simulink library "PES_CZ_FAW"  (Simulink 7.5)
settings: Solver=FixedStepDiscrete  StartTime=0.0  StopTime=10.0  FixedStep=0.01  MaxStep=0.01  RelTol=1e-3
undefined symbols (not defined in the file or in its folder): DiscIntNeverNeededParam, p_DRC_LoPsFilActPwr_s, p_DRC_LoPsFilPwrTi_s, p_DRC_LPFiltIC2_Tau_s, p_DRC_LPFiltIC2_Ts_s, p_DRC_LPFiltIC_Tau_s, p_DRC_LPFiltIC_Ts_s, Slope1, Slope2
libraries: BaseOperationLib_Browser x128, simulink x1
(part 2 of 2)

== system PES_CZ_FAW/Filters/LPFiltICEnRst/UD_EnResetIC ==
  u : Inport
  E : Inport  Port=2
  R : Inport  Port=3
  IC : Inport  Port=4
  Enable : BaseOperationLib_Browser/Signal Routing Changed/Switch  Criteria=u2 ~= 0  Threshold=0  OutMin=[]  OutMax=[]  OutDataType=fixdt(1,16,0)  OutScaling=[]  OutDataTypeStr=Inherit: Inherit via back propagation
  FixPt Data Type Duplicate1 : DataTypeDuplicate  NumInputPorts=4
  UD_Rst_IC : Subsystem
  y : Outport
  wires:
  UD_Rst_IC/1(y) -> y/1, Enable/3, FixPt Data Type Duplicate1/1
  R/1 -> UD_Rst_IC/2(R)
  Enable/1 -> UD_Rst_IC/1(u), FixPt Data Type Duplicate1/3
  u/1 -> Enable/1, FixPt Data Type Duplicate1/4
  IC/1 -> UD_Rst_IC/3(IC), FixPt Data Type Duplicate1/2
  E/1 -> Enable/2

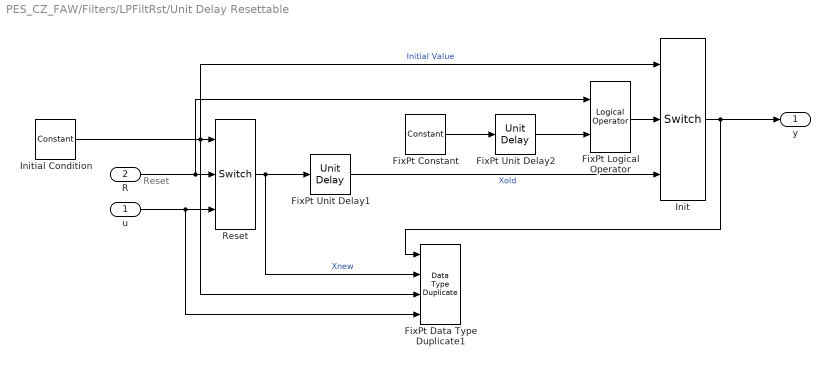
== system PES_CZ_FAW/Filters/LPFiltRst/Unit Delay Resettable ==
  note: Reset
  u : Inport
  R : Inport  Port=2
  FixPt Constant : BaseOperationLib_Browser/Sources&Sinks/Constant  Value=0  OutMin=[]  OutMax=[]  OutDataTypeMode=Specify via dialog  OutDataType=fixdt(0,8,0)  ConRadixGroup=Best Precision: Vector-wise  OutScaling=[]  OutDataTypeStr=fixdt(0,8,0)
  FixPt Data Type Duplicate1 : DataTypeDuplicate  NumInputPorts=4
  FixPt Logical Operator : BaseOperationLib_Browser/Logic Operations Changed/Logical Operator  Operator=OR  Inputs=2  AllPortsSameDT=off  OutDataTypeMode=Specify via dialog  LogicDataType=fixdt(0, 8)  OutDataTypeStr=fixdt(0, 8)
  FixPt Unit Delay1 : BaseOperationLib_Browser/Discrete Unchanged /Unit Delay  X0=0  SampleTime=-1
  FixPt Unit Delay2 : BaseOperationLib_Browser/Discrete Unchanged /Unit Delay  X0=1  SampleTime=-1
  Init : BaseOperationLib_Browser/Signal Routing Changed/Switch  Criteria=u2 ~= 0  Threshold=0  OutMin=[]  OutMax=[]  OutDataType=fixdt(1,16,0)  OutScaling=[]  OutDataTypeStr=Inherit: Inherit via back propagation
  Initial Condition : BaseOperationLib_Browser/Sources&Sinks/Constant  Value=0  OutMin=[]  OutMax=[]  OutDataType=fixdt(1, 16)  ConRadixGroup=Use specified scaling  OutScaling=2^0  OutDataTypeStr=Inherit: Inherit via back propagation
  Reset : BaseOperationLib_Browser/Signal Routing Changed/Switch  Criteria=u2 ~= 0  Threshold=0  OutMin=[]  OutMax=[]  OutDataType=fixdt(1,16,0)  OutScaling=[]  OutDataTypeStr=Inherit: Inherit via back propagation
  y : Outport
  wires:
  Initial Condition/1 -> Reset/1, Init/1, FixPt Data Type Duplicate1/3  "Initial Value"
  u/1 -> FixPt Data Type Duplicate1/4, Reset/3
  Reset/1 -> FixPt Data Type Duplicate1/2, FixPt Unit Delay1/1  "Xnew"
  R/1 -> Reset/2, FixPt Logical Operator/1
  FixPt Constant/1 -> FixPt Unit Delay2/1
  FixPt Unit Delay2/1 -> FixPt Logical Operator/2
  Init/1 -> FixPt Data Type Duplicate1/1, y/1
  FixPt Unit Delay1/1 -> Init/3  "Xold"
  FixPt Logical Operator/1 -> Init/2

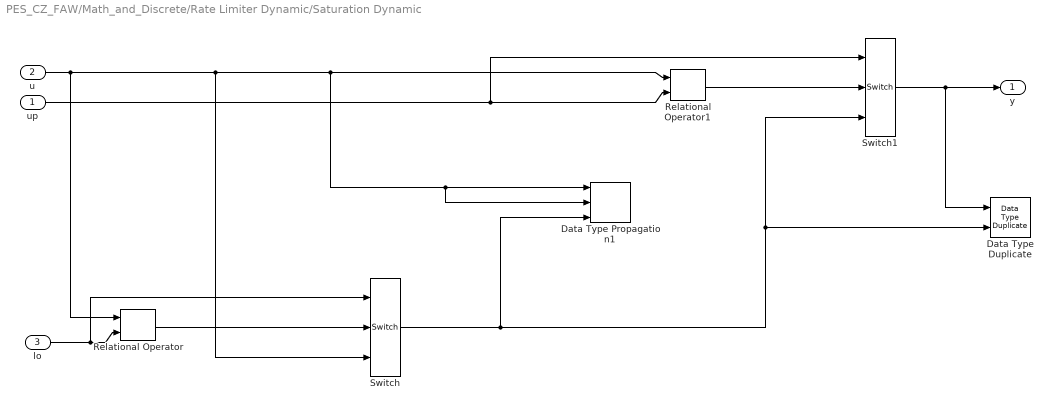
== system PES_CZ_FAW/Math_and_Discrete/Rate Limiter Dynamic/Saturation Dynamic ==
  up : Inport
  u : Inport  Port=2
  lo : Inport  Port=3
  Data Type Duplicate : DataTypeDuplicate
  Data Type Propagation1 : simulink/Signal Attributes/Data Type Propagation  PropDataType=fixdt(1, 16)  IfRefDouble=double  IfRefSingle=single  IsSigned=IsSigned1  NumBitsBase=NumBits1  NumBitsMult=1  NumBitsAdd=0  NumBitsAllowFinal=1:128  PropScaling=2^-10  ValuesUsedBestPrec=[5 -7]  SlopeBase=min([Slope1 Slope2])  SlopeMult=1  SlopeAdd=0  BiasBase=Bias1  BiasMult=1  BiasAdd=0
  Relational Operator : BaseOperationLib_Browser/Logic Operations Changed/Relational Operator  Operator=<  InputSameDT=on  LogicOutDataTypeMode=Specify via dialog  LogicDataType=PDT_Bool  OutDataTypeStr=PDT_Bool
  Relational Operator1 : BaseOperationLib_Browser/Logic Operations Changed/Relational Operator  Operator=>  InputSameDT=on  LogicOutDataTypeMode=Specify via dialog  LogicDataType=PDT_Bool  OutDataTypeStr=PDT_Bool
  Switch : BaseOperationLib_Browser/Signal Routing Changed/Switch  Criteria=u2 ~= 0  Threshold=1  InputSameDT=on  OutMin=[]  OutMax=[]  OutDataType=fixdt(1,16,0)  OutScaling=[]  SaturateOnIntegerOverflow=on
  Switch1 : BaseOperationLib_Browser/Signal Routing Changed/Switch  Criteria=u2 ~= 0  Threshold=1  InputSameDT=on  OutMin=[]  OutMax=[]  OutDataType=fixdt(1,16,0)  OutScaling=[]  SaturateOnIntegerOverflow=on
  y : Outport
  wires:
  up/1 -> Switch1/1, Relational Operator1/2
  u/1 -> Relational Operator/1, Switch/3, Relational Operator1/1, Data Type Propagation1/2, Data Type Propagation1/1
  lo/1 -> Switch/1, Relational Operator/2
  Switch/1 -> Data Type Propagation1/3, Data Type Duplicate/2, Switch1/3
  Switch1/1 -> y/1, Data Type Duplicate/1
  Relational Operator1/1 -> Switch1/2
  Relational Operator/1 -> Switch/2

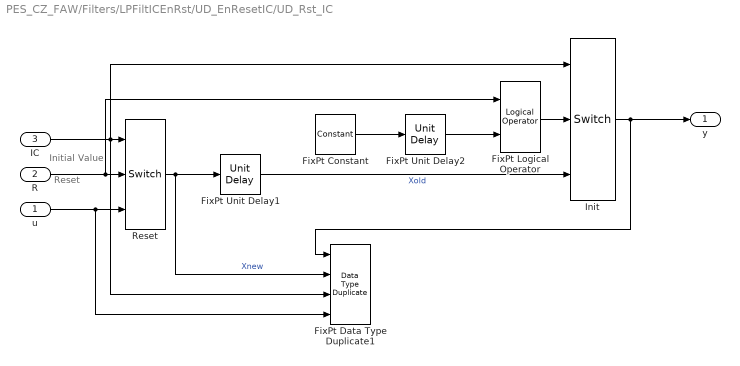
== system PES_CZ_FAW/Filters/LPFiltICEnRst/UD_EnResetIC/UD_Rst_IC ==
  note: Reset
  note: Initial Value
  u : Inport
  R : Inport  Port=2
  IC : Inport  Port=3
  FixPt Constant : BaseOperationLib_Browser/Sources&Sinks/Constant  Value=0  OutMin=[]  OutMax=[]  OutDataTypeMode=Specify via dialog  OutDataType=fixdt(0,8,0)  ConRadixGroup=Best Precision: Vector-wise  OutScaling=[]  OutDataTypeStr=fixdt(0,8,0)
  FixPt Data Type Duplicate1 : DataTypeDuplicate  NumInputPorts=4
  FixPt Logical Operator : BaseOperationLib_Browser/Logic Operations Changed/Logical Operator  Operator=OR  Inputs=2  AllPortsSameDT=off  OutDataTypeMode=Specify via dialog  LogicDataType=fixdt(0, 8)  OutDataTypeStr=fixdt(0, 8)
  FixPt Unit Delay1 : BaseOperationLib_Browser/Discrete Unchanged /Unit Delay  X0=0.0  SampleTime=-1
  FixPt Unit Delay2 : BaseOperationLib_Browser/Discrete Unchanged /Unit Delay  X0=1  SampleTime=-1
  Init : BaseOperationLib_Browser/Signal Routing Changed/Switch  Criteria=u2 ~= 0  Threshold=0  OutMin=[]  OutMax=[]  OutDataType=fixdt(1,16,0)  OutScaling=[]  OutDataTypeStr=Inherit: Inherit via back propagation
  Reset : BaseOperationLib_Browser/Signal Routing Changed/Switch  Criteria=u2 ~= 0  Threshold=0  OutMin=[]  OutMax=[]  OutDataType=fixdt(1,16,0)  OutScaling=[]  OutDataTypeStr=Inherit: Inherit via back propagation
  y : Outport
  wires:
  FixPt Logical Operator/1 -> Init/2
  FixPt Unit Delay1/1 -> Init/3  "Xold"
  Init/1 -> y/1, FixPt Data Type Duplicate1/1
  FixPt Unit Delay2/1 -> FixPt Logical Operator/2
  FixPt Constant/1 -> FixPt Unit Delay2/1
  R/1 -> FixPt Logical Operator/1, Reset/2
  Reset/1 -> FixPt Unit Delay1/1, FixPt Data Type Duplicate1/2  "Xnew"
  u/1 -> Reset/3, FixPt Data Type Duplicate1/4
  IC/1 -> FixPt Data Type Duplicate1/3, Init/1, Reset/1
